simulink subsystem "Subsystem_Motores"  (R2023b)
settings: Solver=VariableStepAuto  StartTime=0.0  StopTime=10.0  RelTol=1e-3
libraries: arduinolib x6, simulink x2
settings Model: Creator=Alberto  LastModifiedBy=Alberto

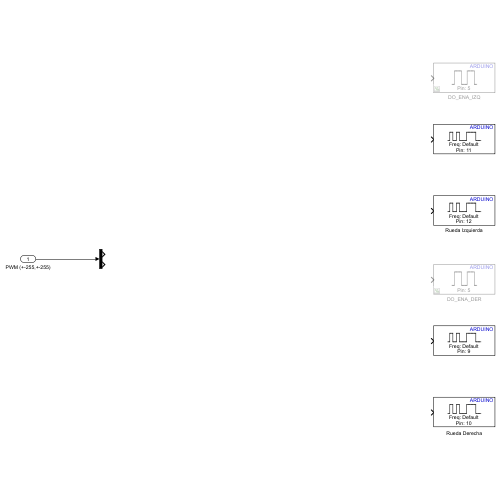
[thumbnail: Simulink's stored preview of the top-level diagram]
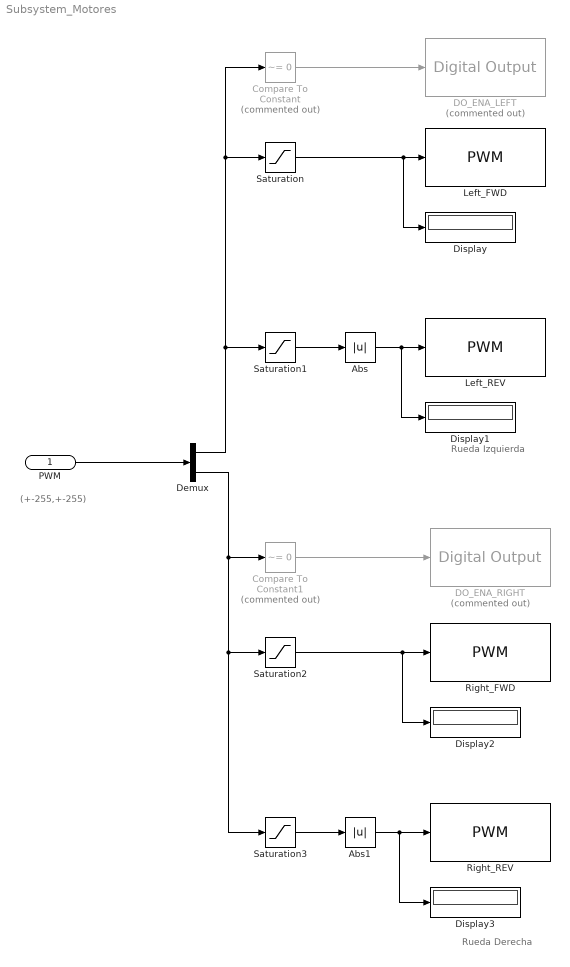
== system Subsystem_Motores ==
  note: (+-255,+-255)
  note: Rueda Izquierda
  note: Rueda Derecha
  PWM : Inport
  Abs : Abs  SaturateOnIntegerOverflow=off
  Abs1 : Abs  SaturateOnIntegerOverflow=off
  Compare To Constant : simulink/Logic and Bit Operations/Compare To Constant  Commented=on  relop=~=  const=0  OutDataTypeStr=boolean
  Compare To Constant1 : simulink/Logic and Bit Operations/Compare To Constant  Commented=on  relop=~=  const=0  OutDataTypeStr=boolean
  DO_ENA_LEFT : arduinolib/Digital Output  Commented=on  pinNumber=8  Direction=output  blockPlatform=arduino
  DO_ENA_RIGHT : arduinolib/Digital Output  Commented=on  pinNumber=13  Direction=output  blockPlatform=arduino
  Demux : Demux  Outputs=2
  Display{,1..3} (4 alike) : Display
  Left_FWD : arduinolib/PWM  pinNumber=9  frequencyType=Default  desiredFrequency=490.2  achievableFrequency=490.2
  Left_REV : arduinolib/PWM  pinNumber=10  frequencyType=Default  desiredFrequency=490.2  achievableFrequency=490.2
  Right_FWD : arduinolib/PWM  pinNumber=11  frequencyType=Default  desiredFrequency=490.2  achievableFrequency=490.2
  Right_REV : arduinolib/PWM  pinNumber=12  frequencyType=Default  desiredFrequency=490.2  achievableFrequency=490.2
  Saturation : Saturate  UpperLimit=255  LowerLimit=1
  Saturation1 : Saturate  UpperLimit=0  LowerLimit=-255
  Saturation2 : Saturate  UpperLimit=255  LowerLimit=1
  Saturation3 : Saturate  UpperLimit=0  LowerLimit=-255
  wires:
  Demux/1 -> Compare To Constant/1, Saturation/1, Saturation1/1
  Compare To Constant/1 -> DO_ENA_LEFT/1
  Abs/1 -> Display1/1, Left_REV/1
  Compare To Constant1/1 -> DO_ENA_RIGHT/1
  Abs1/1 -> Right_REV/1, Display3/1
  Demux/2 -> Compare To Constant1/1, Saturation2/1, Saturation3/1
  Saturation/1 -> Left_FWD/1, Display/1
  Saturation1/1 -> Abs/1
  Saturation3/1 -> Abs1/1
  Saturation2/1 -> Right_FWD/1, Display2/1
  PWM/1 -> Demux/1
